simulink model "ex11_2"  (R2020b)
settings: Solver=VariableStepAuto  StartTime=0.0  StopTime=0.033  RelTol=1e-3
libraries: powerlib x12, powerlib_meascontrol x5
settings Model: Creator=Asus  LastModifiedBy=macbook
settings DataIOCC: ReturnWorkspaceOutputs=off
settings DebuggingCC: ArithmeticOperatorsInVariantConditions=warning
settings SFSimCC: SimUseLocalCustomCode=off  CustomCodeUndefinedFunction=UseInterfaceOnly
settings RTWCC: RTWUseLocalCustomCode=off

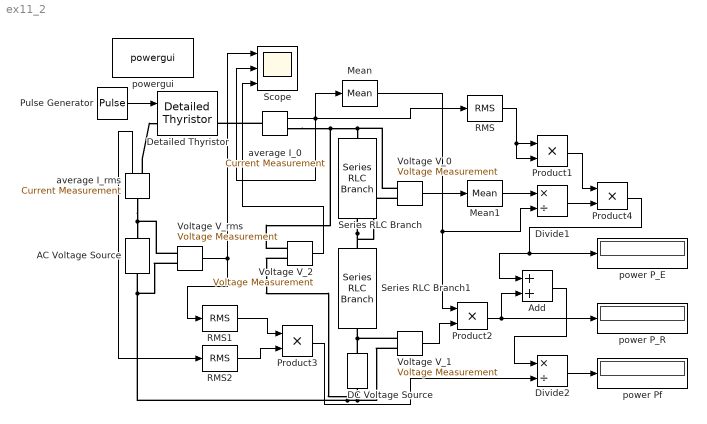
== system ex11_2 ==
  AC Voltage Source : powerlib/Electrical Sources/AC Voltage Source  Amplitude=120*sqrt(2)  Phase=0  Frequency=60  SampleTime=0  Measurements=None  BusType=swing  Pref=10e3  Qref=0  Qmin=-inf  Qmax=+inf
  Add : Sum
  DC Voltage Source : powerlib/Electrical Sources/DC Voltage Source  Amplitude=48  Measurements=None
  Detailed Thyristor : powerlib/Power Electronics/Detailed Thyristor  Ron=0.001  Lon=1e-3  Vf=0.8  IL=0.1  Tq=100e-6  IC=0.549  Rs=100  Cs=250e-9  Measurements=on
      settings: SourceProductBaseCode=PS
  Divide1 : Product  Inputs=*/
  Divide2 : Product  Inputs=*/
  Mean : powerlib_meascontrol/Measurements/Mean  Freq=60  Vinit=0  Ts=0
  Mean1 : powerlib_meascontrol/Measurements/Mean  Freq=60  Vinit=0  Ts=0
  Product{1..4} (4 alike) : Product
  Pulse Generator : DiscretePulseGenerator  PulseType=Time based  Period=0.01666  PulseWidth=10  PhaseDelay=30/(180*120)
  RMS : powerlib_meascontrol/Measurements/RMS  TrueRMS=on  Freq=60  RMSInit=120  Ts=0
  RMS1 : powerlib_meascontrol/Measurements/RMS  TrueRMS=on  Freq=60  RMSInit=120  Ts=0
  RMS2 : powerlib_meascontrol/Measurements/RMS  TrueRMS=on  Freq=60  RMSInit=120  Ts=0
  Scope : Scope  NumInputPorts=3
  Series RLC Branch : powerlib/Elements/Series RLC Branch  LConnTagsString=__new0  RConnTagsString=__new0  BranchType=R  Resistance=12  Inductance=1e-3  SetiL0=off  InitialCurrent=0  Capacitance=1e-6  Setx0=off  InitialVoltage=0  Measurements=None
  Series RLC Branch1 : powerlib/Elements/Series RLC Branch  LConnTagsString=__new0  RConnTagsString=__new0  BranchType=L  Resistance=30  Inductance=0.1  SetiL0=off  InitialCurrent=0  Capacitance=1e-6  Setx0=off  InitialVoltage=0  Measurements=None
  Voltage V_0 : powerlib/Measurements/Voltage Measurement  PhasorSimulation=off  OutputType=Complex  PSBequivalent=0
  Voltage V_1 : powerlib/Measurements/Voltage Measurement  PhasorSimulation=off  OutputType=Complex  PSBequivalent=0
  Voltage V_2 : powerlib/Measurements/Voltage Measurement  PhasorSimulation=off  OutputType=Complex  PSBequivalent=0
  Voltage V_rms : powerlib/Measurements/Voltage Measurement  PhasorSimulation=off  OutputType=Complex  PSBequivalent=0
  "average I_0 " : powerlib/Measurements/Current Measurement  PhasorSimulation=off  OutputType=Complex  PSBequivalent=0
  "average I_rms " : powerlib/Measurements/Current Measurement  PhasorSimulation=off  OutputType=Complex  PSBequivalent=0
  power P_E : Display
  power P_R : Display
  "power Pf " : Display
  powergui : powerlib/powergui  Priority=1  SimulationMode=Continuous  SampleTime=50e-6  frequency=60  Iterations=50  frequencyindice=0  Pbase=100e6  ErrMax=1e-4  UnitsV=kV  UnitsW=MW  buscounter=0  FunctionMessages=off  echomessages=off  EnableUseOfTLC=off  CurrentSourceSwitches=off  DisableSnubberDevices=off  DisableRonSwitches=off  DisableVfSwitches=off  DisplayEquations=off  AutomaticDiscreteSolvers=off  SolverType=Tustin/Backward Euler (TBE)  Interpol=off  ExternalGateDelay=off  methode=off  Ts=100  x0status=blocks  SPID=on  SwTol=0  HookPort=off  NonlinearTolerance=1e-4  nMaxIteration=100  ContinueOnMaxIteration=off  RestoreLinks=warning  ResistiveCurrentMeasurement=off  Frange=[0:2:500]  Ylog=off  Xlog=on  ShowGrid=off  save=off  variable=ZData  structure=0  ZoomFFT=off  StartTime=0.0  cycles=1  DisplayStyle=1  fundamental=60  FreqAxis=off  MaxFrequency=1000  frequencyindicesteady=1  RmsSteady=1  display=off
  wires:
  Voltage V_rms/1 -> RMS1/1, Scope/1
  Pulse Generator/1 -> Detailed Thyristor/1
  "average I_0 "/1 -> Mean/1, Scope/2, RMS/1
  Voltage V_0/1 -> Mean1/1
  Mean/1 -> Product2/1, Divide1/2
  "average I_rms "/1 -> RMS2/1
  RMS1/1 -> Product3/1
  RMS2/1 -> Product3/2
  Voltage V_1/1 -> Product2/2
  Product2/1 -> Add/2, power P_R/1
  Mean1/1 -> Divide1/1
  Product4/1 -> power P_E/1, Add/1
  Product1/1 -> Product4/1
  Divide1/1 -> Product4/2
  RMS/1 -> Product1/2, Product1/1
  Add/1 -> Divide2/1
  Divide2/1 -> "power Pf "/1
  Product3/1 -> Divide2/2
  Voltage V_2/1 -> Scope/3
  connections:
  Voltage V_rms/LConn2 -- Voltage V_2/LConn2 -- DC Voltage Source/LConn1 -- Voltage V_1/LConn2 -- AC Voltage Source/LConn1
  "average I_0 "/RConn1 -- Voltage V_0/LConn1 -- Series RLC Branch/LConn1 -- Voltage V_2/LConn1
  AC Voltage Source/RConn1 -- "average I_rms "/LConn1 -- Voltage V_rms/LConn1
  Series RLC Branch1/LConn1 -- Voltage V_0/LConn2 -- Series RLC Branch/RConn1
  "average I_0 "/LConn1 -- Detailed Thyristor/RConn1
  "average I_rms "/RConn1 -- Detailed Thyristor/LConn1
  DC Voltage Source/RConn1 -- Series RLC Branch1/RConn1 -- Voltage V_1/LConn1
